simulink model "HalfCar_Model"  (R2018b)
settings: Solver=VariableStepAuto  StartTime=0.0  StopTime=14  RelTol=1e-3
values from neighbouring files (symbols this model uses):
  a = 1.25    [SetCoefficients_FC.m]
  amplitude = 0.01    [SetCoefficients_FC.m]
  b = 1.4    [SetCoefficients_FC.m]
  csc = 600    [SetCoefficients_FC.m]
  cse = 1200    [SetCoefficients_FC.m]
  delay = (a+b)/v    [setSpeed.m]
  Fre_r = Fre*2*pi    [setSpeed.m]
  g = 9.81    [SetCoefficients_FC.m]
  HumpHight = 2    [SetCoefficients_FC.m]
  HumpLegnth = 20    [SetCoefficients_FC.m]
  I = 600    [SetCoefficients_FC.m]
  ks =     [SetCoefficients.m]    (also in SetCoefficients_FC.m = 20000)
  ksstiff = 4e5    (= 400000)    [SetCoefficients_FC.m]
  kt =     [SetCoefficients.m]    (also in SetCoefficients_FC.m = 140000)
  m2 =     [SetCoefficients.m]    (also in SetCoefficients_FC.m = 20)
  mb = 1000    [SetCoefficients_FC.m]
  v = 10    [SetCoefficients_FC.m]
  x1 = 0.2    [SetCoefficients_FC.m]
  x2 = 0.25    [SetCoefficients_FC.m]
settings Model: Creator=joebe  LastModifiedBy=joebe

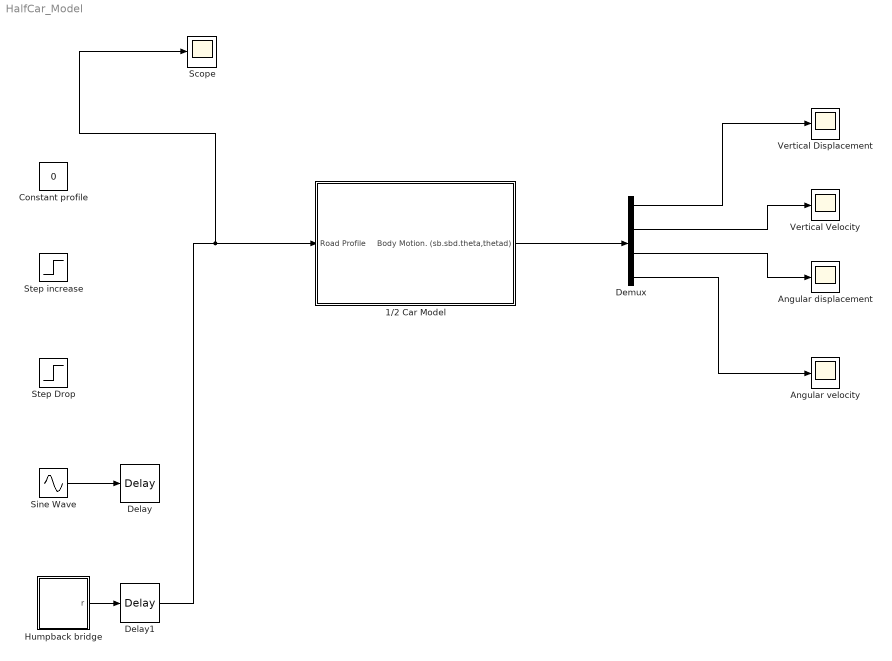
== system HalfCar_Model ==
  1/2 Car Model : Subsystem
  Angular displacement : Scope
  Angular velocity : Scope
  Constant profile : Constant  Value=0
  Delay : TransportDelay  BufferSize=3072
  Delay1 : TransportDelay  BufferSize=3072
  Demux : Demux
  Humpback bridge : Subsystem  mask{h=HumpHight, L=HumpLegnth, v=v}
      mask prompts: h "humpback height (m)"; L "humpback length (m)"; v "vehicle speed (m/s)"
  Scope : Scope
  Sine Wave : Sin  Amplitude=amplitude  Frequency=Fre_r  SampleTime=0
  Step Drop : Step  Time=2  After=-2  SampleTime=0
  Step increase : Step  Time=2  SampleTime=0
  Vertical Displacement : Scope
  Vertical Velocity : Scope
  wires:
  1/2 Car Model/1(Body Motion. (sb.sbd.theta,thetad)) -> Demux/1
  Demux/1 -> Vertical Displacement/1
  Demux/2 -> Vertical Velocity/1
  Demux/3 -> Angular displacement/1
  Demux/4 -> Angular velocity/1
  Sine Wave/1 -> Delay/1
  Humpback bridge/1(r) -> Delay1/1
  Delay1/1 -> Scope/1, 1/2 Car Model/1(Road Profile)

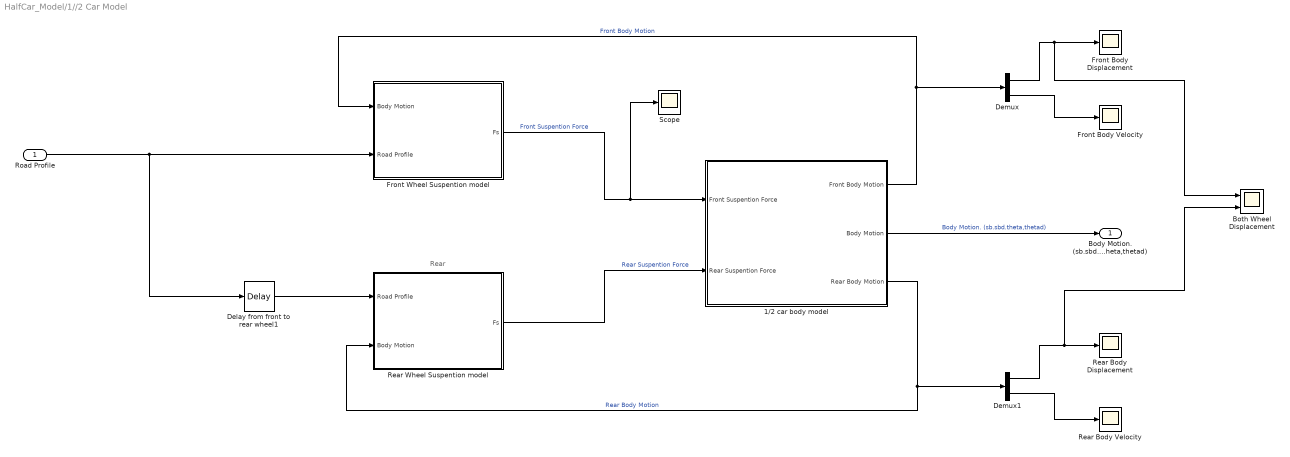
== system HalfCar_Model/1//2 Car Model ==
  note: Rear
  Road Profile : Inport
  1/2 car body model : Subsystem
  Both Wheel Displacement : Scope  NumInputPorts=2
  Delay from front to rear wheel1 : TransportDelay  DelayTime=delay  BufferSize=3072
  Demux : Demux  Outputs=2
  Demux1 : Demux  Outputs=2
  Front Body Displacement : Scope
  Front Body Velocity : Scope
  Front Wheel Suspention model : Subsystem
  Rear Body Displacement : Scope
  Rear Body Velocity : Scope
  Rear Wheel Suspention model : Subsystem
  Scope : Scope
  Body Motion. (sb.sbd.theta,thetad) : Outport
  wires:
  1/2 car body model/3(Rear Body Motion) -> Demux1/1, Rear Wheel Suspention model/2(Body Motion)  "Rear Body Motion"
  Demux1/2 -> Rear Body Velocity/1
  Demux/2 -> Front Body Velocity/1
  Road Profile/1 -> Delay from front to rear wheel1/1, Front Wheel Suspention model/2(Road Profile)
  Demux/1 -> Both Wheel Displacement/1, Front Body Displacement/1
  Demux1/1 -> Both Wheel Displacement/2, Rear Body Displacement/1
  Front Wheel Suspention model/1(Fs) -> Scope/1, 1/2 car body model/1(Front Suspention Force)  "Front Suspention Force"
  Rear Wheel Suspention model/1(Fs) -> 1/2 car body model/2(Rear Suspention Force)  "Rear Suspention Force"
  1/2 car body model/1(Front Body Motion) -> Demux/1, Front Wheel Suspention model/1(Body Motion)  "Front Body Motion"
  1/2 car body model/2(Body Motion) -> Body Motion. (sb.sbd.theta,thetad)/1  "Body Motion. (sb.sbd.theta,thetad)"
  Delay from front to rear wheel1/1 -> Rear Wheel Suspention model/1(Road Profile)

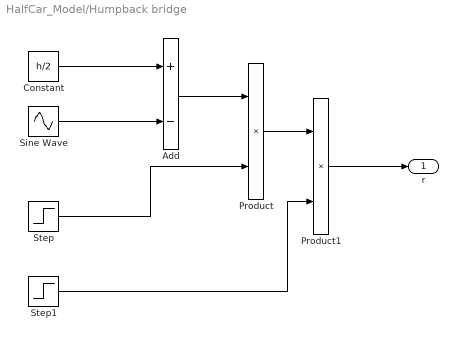
== system HalfCar_Model/Humpback bridge ==
  Add : Sum  Inputs=+-
  Constant : Constant  Value=h/2
  Product : Product
  Product1 : Product
  Sine Wave : Sin  Amplitude=h/2  Frequency=2*pi*v/L  Phase=pi/2  SampleTime=0
  Step : Step  Time=0  SampleTime=0
  Step1 : Step  Time=L/v  Before=1  After=0  SampleTime=0
  r : Outport
  wires:
  Constant/1 -> Add/1
  Sine Wave/1 -> Add/2
  Add/1 -> Product/1
  Step/1 -> Product/2
  Product/1 -> Product1/1
  Step1/1 -> Product1/2
  Product1/1 -> r/1

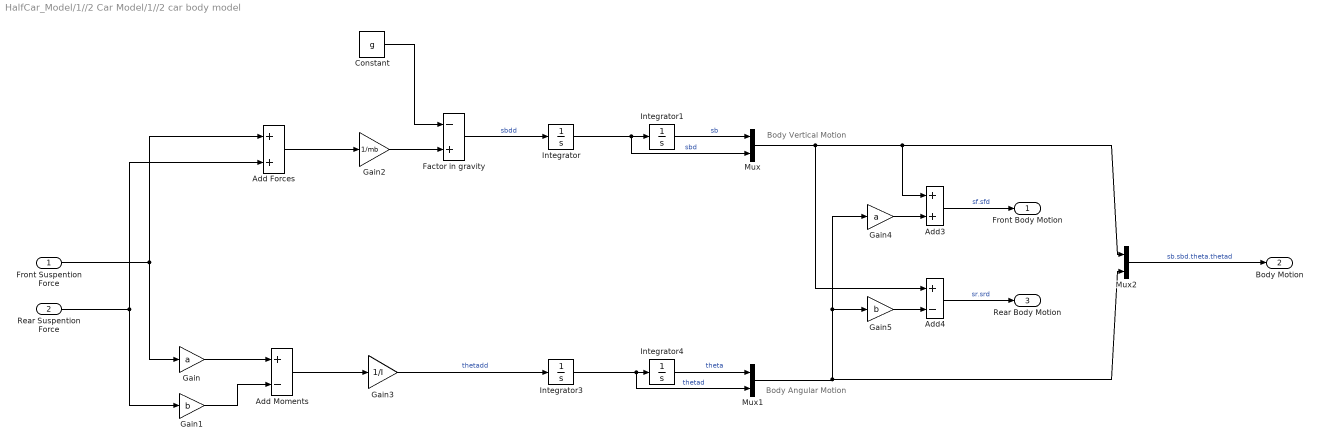
== system HalfCar_Model/1//2 Car Model/1//2 car body model ==
  note: Body Angular Motion
  note: Body Vertical Motion
  Front Suspention Force : Inport
  Rear Suspention Force : Inport  Port=2
  Add Forces : Sum
  Add Moments : Sum  Inputs=+-
  Add3 : Sum
  Add4 : Sum  Inputs=+-
  Constant : Constant  Value=g
  Factor in gravity : Sum  Inputs=-+
  Gain : Gain  Gain=a
  Gain1 : Gain  Gain=b
  Gain2 : Gain  Gain=1/mb
  Gain3 : Gain  Gain=1/I
  Gain4 : Gain  Gain=a
  Gain5 : Gain  Gain=b
  Integrator : Integrator
  Integrator1 : Integrator  InitialCondition=-0.142
  Integrator3 : Integrator
  Integrator4 : Integrator  InitialCondition=-6e-3
  Mux : Mux  Inputs=2
  Mux1 : Mux  Inputs=2
  Mux2 : Mux  Inputs=2
  Front Body Motion : Outport
  Body Motion : Outport  Port=2
  Rear Body Motion : Outport  Port=3
  wires:
  Add Forces/1 -> Gain2/1
  Mux1/1 -> Gain4/1, Gain5/1, Mux2/2
  Integrator3/1 -> Mux1/2, Integrator4/1  "thetad"
  Add Moments/1 -> Gain3/1
  Gain3/1 -> Integrator3/1  "thetadd"
  Mux2/1 -> Body Motion/1  "sb.sbd.theta.thetad"
  Gain2/1 -> Factor in gravity/2
  Mux/1 -> Add4/1, Add3/1, Mux2/1
  Gain4/1 -> Add3/2
  Gain/1 -> Add Moments/1
  Integrator4/1 -> Mux1/1  "theta"
  Integrator/1 -> Mux/2, Integrator1/1  "sbd"
  Rear Suspention Force/1 -> Add Forces/2, Gain1/1
  Front Suspention Force/1 -> Gain/1, Add Forces/1
  Integrator1/1 -> Mux/1  "sb"
  Gain1/1 -> Add Moments/2
  Add3/1 -> Front Body Motion/1  "sf.sfd"
  Gain5/1 -> Add4/2
  Constant/1 -> Factor in gravity/1
  Factor in gravity/1 -> Integrator/1  "sbdd"
  Add4/1 -> Rear Body Motion/1  "sr.srd"

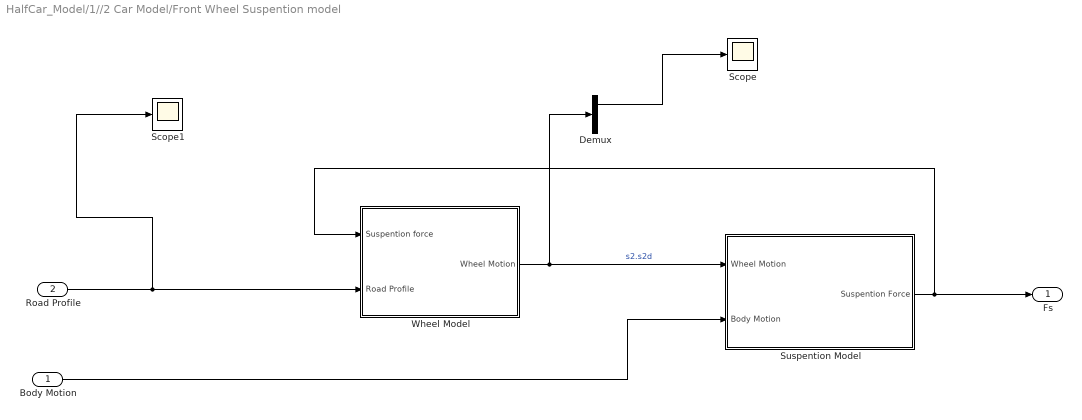
== system HalfCar_Model/1//2 Car Model/Front Wheel Suspention model ==
  Body Motion : Inport
  Road Profile : Inport  Port=2
  Demux : Demux  Outputs=2
  Scope : Scope
  Scope1 : Scope
  Suspention Model : Subsystem
  Wheel Model : Subsystem
  Fs : Outport
  wires:
  Wheel Model/1(Wheel Motion) -> Demux/1, Suspention Model/1(Wheel Motion)  "s2.s2d"
  Road Profile/1 -> Scope1/1, Wheel Model/2(Road Profile)
  Suspention Model/1(Suspention Force) -> Fs/1, Wheel Model/1(Suspention force)
  Body Motion/1 -> Suspention Model/2(Body Motion)
  Demux/1 -> Scope/1

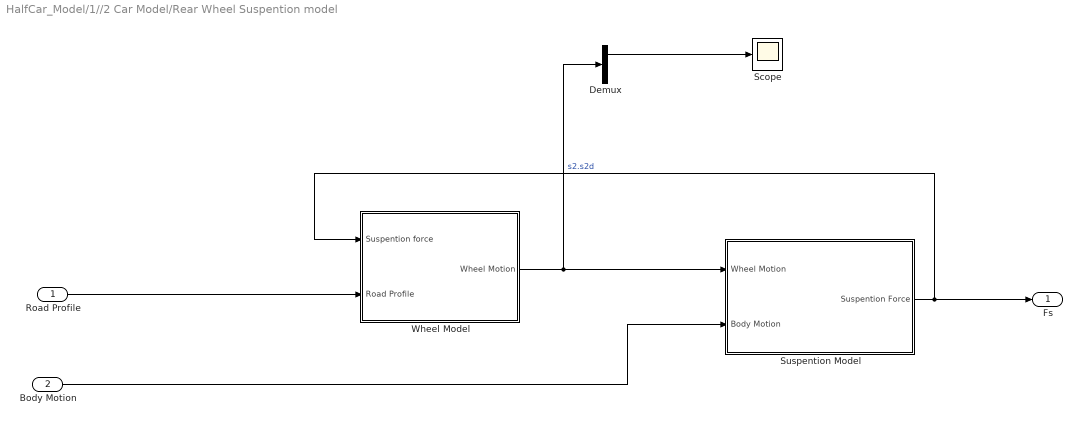
== system HalfCar_Model/1//2 Car Model/Rear Wheel Suspention model ==
  Road Profile : Inport
  Body Motion : Inport  Port=2
  Demux : Demux  Outputs=2
  Scope : Scope
  Suspention Model : Subsystem
  Wheel Model : Subsystem
  Fs : Outport
  wires:
  Wheel Model/1(Wheel Motion) -> Demux/1, Suspention Model/1(Wheel Motion)  "s2.s2d"
  Road Profile/1 -> Wheel Model/2(Road Profile)
  Suspention Model/1(Suspention Force) -> Fs/1, Wheel Model/1(Suspention force)
  Body Motion/1 -> Suspention Model/2(Body Motion)
  Demux/1 -> Scope/1

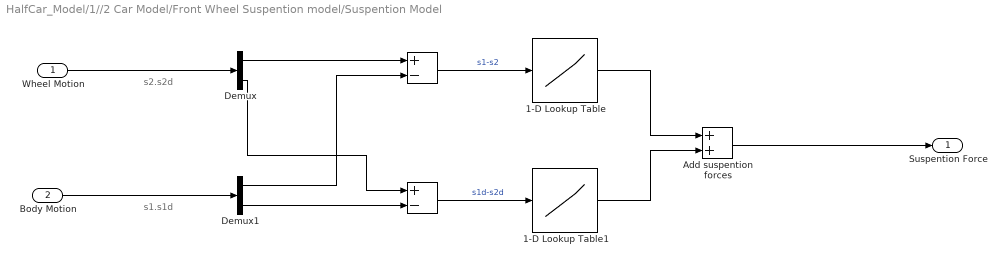
== system HalfCar_Model/1//2 Car Model/Front Wheel Suspention model/Suspention Model ==
  note: s1.s1d
  note: s2.s2d
  Wheel Motion : Inport
  Body Motion : Inport  Port=2
  " " : Sum  Inputs=+-
  " " : Sum  Inputs=+-
  1-D Lookup Table : Lookup_n-D  NumberOfTableDimensions=1  BreakpointsForDimension1=[-x2 -x1 x1 x2]  Table=[-(ksstiff*(x2-x1)+ks*x1) -x1*ks x1*ks (ksstiff*(x2-x1)+ks*x1)]  InternalRulePriority=Speed  RndMeth=Simplest  InputSameDT=on
  1-D Lookup Table1 : Lookup_n-D  NumberOfTableDimensions=1  BreakpointsForDimension1=[-10 0 10]  Table=[-10*cse 0 10*csc]  InternalRulePriority=Speed  RndMeth=Simplest  InputSameDT=on
  Add suspention forces : Sum
  Demux : Demux  Outputs=2
  Demux1 : Demux  Outputs=2
  Suspention Force : Outport
  wires:
  Demux1/2 -> " "/2
  " "/1 -> 1-D Lookup Table/1  "s1-s2"
  Demux1/1 -> " "/2
  1-D Lookup Table1/1 -> Add suspention forces/2
  1-D Lookup Table/1 -> Add suspention forces/1
  Demux/1 -> " "/1
  Demux/2 -> " "/1
  Body Motion/1 -> Demux1/1
  " "/1 -> 1-D Lookup Table1/1  "s1d-s2d"
  Add suspention forces/1 -> Suspention Force/1
  Wheel Motion/1 -> Demux/1

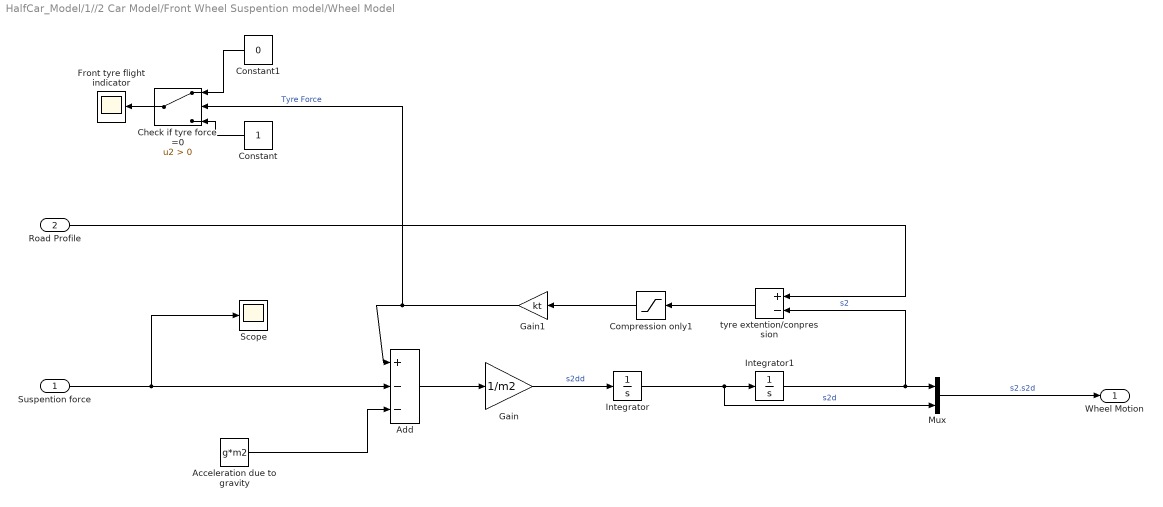
== system HalfCar_Model/1//2 Car Model/Front Wheel Suspention model/Wheel Model ==
  Suspention force : Inport
  Road Profile : Inport  Port=2
  Acceleration due to gravity : Constant  Value=g*m2
  Add : Sum  Inputs=+--
  Check if tyre force =0 : Switch  Criteria=u2 > Threshold
  Compression only1 : Saturate  UpperLimit=inf  LowerLimit=0
  Constant : Constant
  Constant1 : Constant  Value=0
  Front tyre flight indicator : Scope
  Gain : Gain  Gain=1/m2
  Gain1 : Gain  Gain=kt
  Integrator : Integrator
  Integrator1 : Integrator  InitialCondition=-0.02
  Mux : Mux  Inputs=2
  Scope : Scope
  tyre extention/conpression : Sum  Inputs=+-
  Wheel Motion : Outport
  wires:
  Integrator1/1 -> Mux/1, tyre extention/conpression/2  "s2"
  Integrator/1 -> Mux/2, Integrator1/1  "s2d"
  Add/1 -> Gain/1
  Gain1/1 -> Check if tyre force =0/2, Add/1  "Tyre Force"
  Road Profile/1 -> tyre extention/conpression/1
  Mux/1 -> Wheel Motion/1  "s2.s2d"
  Acceleration due to gravity/1 -> Add/3
  Suspention force/1 -> Scope/1, Add/2
  Gain/1 -> Integrator/1  "s2dd"
  tyre extention/conpression/1 -> Compression only1/1
  Compression only1/1 -> Gain1/1
  Check if tyre force =0/1 -> Front tyre flight indicator/1
  Constant1/1 -> Check if tyre force =0/1
  Constant/1 -> Check if tyre force =0/3

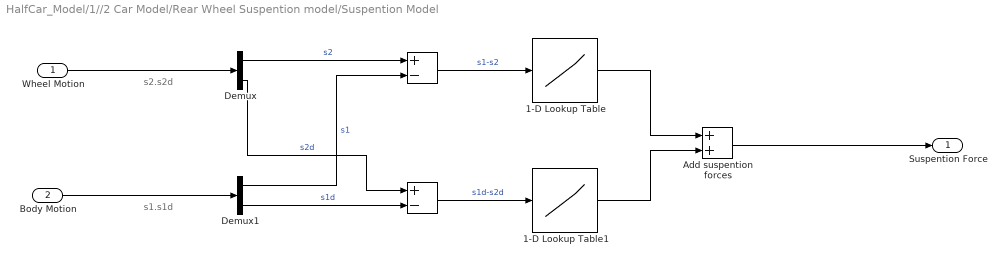
== system HalfCar_Model/1//2 Car Model/Rear Wheel Suspention model/Suspention Model ==
  note: s1.s1d
  note: s2.s2d
  Wheel Motion : Inport
  Body Motion : Inport  Port=2
  " " : Sum  Inputs=+-
  " " : Sum  Inputs=+-
  1-D Lookup Table : Lookup_n-D  NumberOfTableDimensions=1  BreakpointsForDimension1=[-x2 -x1 x1 x2]  Table=[-(ksstiff*(x2-x1)+ks*x1) -x1*ks x1*ks (ksstiff*(x2-x1)+ks*x1)]  InternalRulePriority=Speed  RndMeth=Simplest  InputSameDT=on
  1-D Lookup Table1 : Lookup_n-D  NumberOfTableDimensions=1  BreakpointsForDimension1=[-10 0 10]  Table=[-10*cse 0 10*csc]  InternalRulePriority=Speed  RndMeth=Simplest  InputSameDT=on
  Add suspention forces : Sum
  Demux : Demux  Outputs=2
  Demux1 : Demux  Outputs=2
  Suspention Force : Outport
  wires:
  Demux1/2 -> " "/2  "s1d"
  " "/1 -> 1-D Lookup Table/1  "s1-s2"
  Demux1/1 -> " "/2  "s1"
  1-D Lookup Table1/1 -> Add suspention forces/2
  1-D Lookup Table/1 -> Add suspention forces/1
  Demux/1 -> " "/1  "s2"
  Demux/2 -> " "/1  "s2d"
  Body Motion/1 -> Demux1/1
  " "/1 -> 1-D Lookup Table1/1  "s1d-s2d"
  Add suspention forces/1 -> Suspention Force/1
  Wheel Motion/1 -> Demux/1

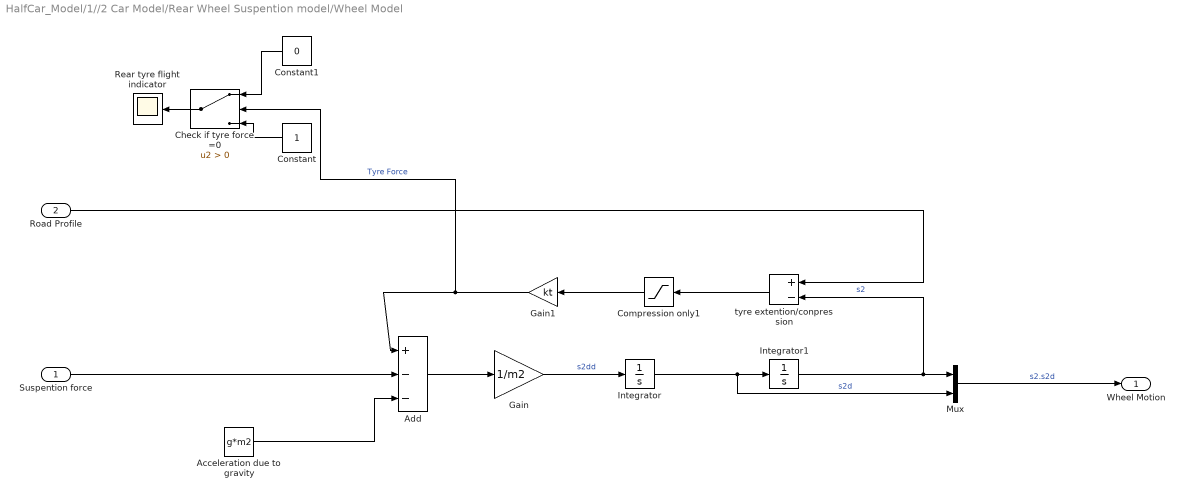
== system HalfCar_Model/1//2 Car Model/Rear Wheel Suspention model/Wheel Model ==
  Suspention force : Inport
  Road Profile : Inport  Port=2
  Acceleration due to gravity : Constant  Value=g*m2
  Add : Sum  Inputs=+--
  Check if tyre force =0 : Switch  Criteria=u2 > Threshold
  Compression only1 : Saturate  UpperLimit=inf  LowerLimit=0
  Constant : Constant
  Constant1 : Constant  Value=0
  Gain : Gain  Gain=1/m2
  Gain1 : Gain  Gain=kt
  Integrator : Integrator
  Integrator1 : Integrator  InitialCondition=-0.018
  Mux : Mux  Inputs=2
  Rear tyre flight indicator : Scope
  tyre extention/conpression : Sum  Inputs=+-
  Wheel Motion : Outport
  wires:
  Integrator1/1 -> tyre extention/conpression/2, Mux/1  "s2"
  Integrator/1 -> Mux/2, Integrator1/1  "s2d"
  Add/1 -> Gain/1
  Gain1/1 -> Check if tyre force =0/2, Add/1  "Tyre Force"
  Road Profile/1 -> tyre extention/conpression/1
  Mux/1 -> Wheel Motion/1  "s2.s2d"
  Acceleration due to gravity/1 -> Add/3
  Suspention force/1 -> Add/2
  Gain/1 -> Integrator/1  "s2dd"
  tyre extention/conpression/1 -> Compression only1/1
  Compression only1/1 -> Gain1/1
  Constant/1 -> Check if tyre force =0/3
  Check if tyre force =0/1 -> Rear tyre flight indicator/1
  Constant1/1 -> Check if tyre force =0/1
